simulink model "ClaseControl_30_01"  (R2021b)
settings: Solver=VariableStepAuto  StartTime=0.0  StopTime=10  RelTol=1e-3
settings Model: Creator=Duván Ramírez Lotta  LastModifiedBy=Duván Ramírez Lotta

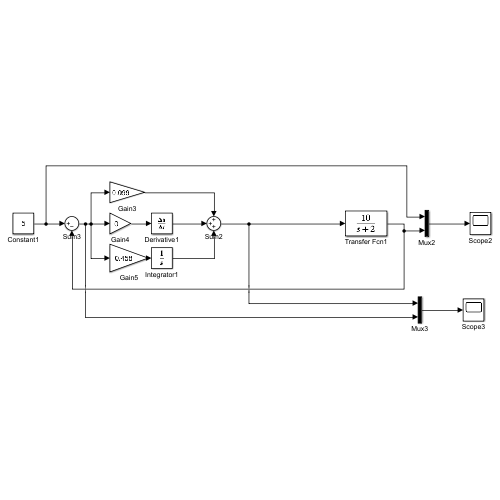
[thumbnail: Simulink's stored preview of the top-level diagram]
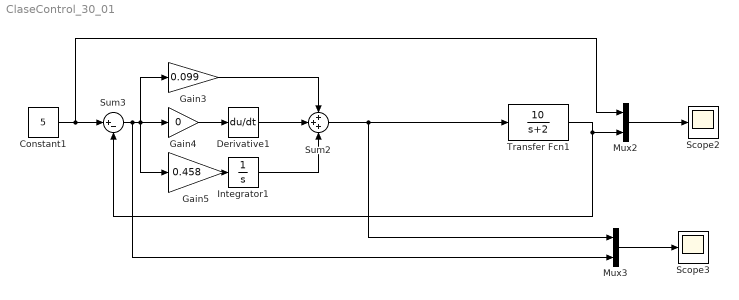
== system ClaseControl_30_01 ==
  Constant1 : Constant  Value=5
  Derivative1 : Derivative
  Gain3 : Gain  Gain=0.099
  Gain4 : Gain  Gain=0
  Gain5 : Gain  Gain=0.458
  Integrator1 : Integrator
  Mux2 : Mux  Inputs=2
  Mux3 : Mux  Inputs=2
  Scope2 : Scope
  Scope3 : Scope
  Sum2 : Sum  Inputs=+++
  Sum3 : Sum  Inputs=|+-
  Transfer Fcn1 : TransferFcn  Numerator=10  Denominator=[1 2]
  wires:
  Integrator1/1 -> Sum2/3
  Constant1/1 -> Mux2/1, Sum3/1
  Derivative1/1 -> Sum2/2
  Sum3/1 -> Mux3/2, Gain5/1, Gain3/1, Gain4/1
  Mux3/1 -> Scope3/1
  Gain4/1 -> Derivative1/1
  Gain3/1 -> Sum2/1
  Gain5/1 -> Integrator1/1
  Mux2/1 -> Scope2/1
  Transfer Fcn1/1 -> Mux2/2, Sum3/2
  Sum2/1 -> Mux3/1, Transfer Fcn1/1
